simulink model "flyWheel_ss"  (R2018b)
settings: Solver=VariableStepAuto  StartTime=0.0  StopTime=10.0  RelTol=1e-3
settings Model: Creator=ROG  LastModifiedBy=ROG

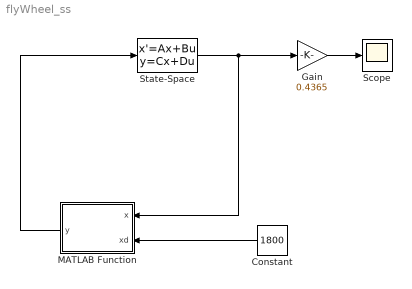
== system flyWheel_ss ==
  Constant : Constant  Value=1800
  Gain : Gain  Gain=0.4365
  MATLAB Function : MATLAB Function  TreatAsAtomicUnit=on
  Scope : Scope
  State-Space : StateSpace  A=-2.1226  D=0  InitialCondition=0
  wires:
  State-Space/1 -> MATLAB Function/1(x), Gain/1
  MATLAB Function/1(y) -> State-Space/1
  Gain/1 -> Scope/1
  Constant/1 -> MATLAB Function/2(xd)

== matlab function flyWheel_ss/MATLAB Function ==
  data: x input; y output; xd input
function y = fcn(x, xd)
A = [-2.1226];
B = [1];

%%
S = [1];
Q = [1];
R = 0.1;
%%
[Aa, Ba, Qa, Sa, R, ud] = ia_LQR(A, B, Q, R, S, xd);
[F] = F1_LQR_Gain(Aa, Ba, Qa, R, Sa);

xa = [x;xd];

u = -F * (xa) + ud;

y = u;
